simulink model "fskmodelo"  (R2015a)
settings: Solver=ode45  StartTime=0.0  StopTime=10.0  RelTol=1e-3
libraries: commdigbbndfm2 x2, commchan3 x1, commrandsrc2 x1, commsink2 x1
settings Model: Creator=francisco  LastModifiedBy=francisco

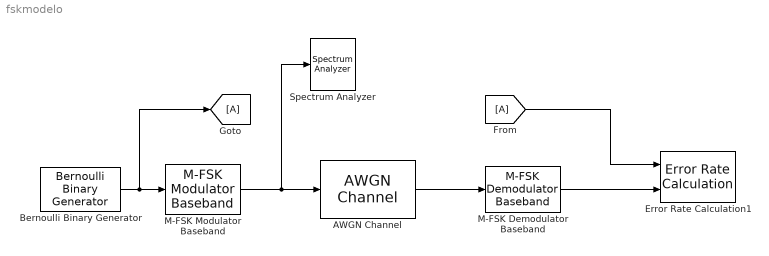
== system fskmodelo ==
  AWGN Channel : commchan3/AWGN Channel  InputProcessing=Columns as channels (frame based)  seed=67  noiseMode="Signal to noise ratio  (Eb/No)"  EbNodB=15  EsNodB=10  SNRdB=10  bitsPerSym=1  Ps=1  Tsym=1  variance=1
  Bernoulli Binary Generator : commrandsrc2/Bernoulli Binary Generator  P=0.5  seed=61  Ts=0.01  frameBased=off  sampPerFrame=1  orient=off  outDataType=double
  Error Rate Calculation1 : commsink2/Error Rate Calculation  N=0  st_delay=0  cp_mode=Entire frame  subframe=[]  PMode=Workspace  WsName=ErrorVec  RsMode2=off  stop=off  numErr=100  maxBits=1e6
  M-FSK Demodulator Baseband : commdigbbndfm2/M-FSK Demodulator Baseband  M=4  OutType=Integer  Dec=Gray  freqSep=100  numSamp=17  RateOptions=Enforce single-rate processing  outDataType=double
  M-FSK Modulator Baseband : commdigbbndfm2/M-FSK Modulator Baseband  M=4  InType=Integer  Enc=Gray  freqSep=100  phaseType=Continuous  numSamp=17  RateOptions=Enforce single-rate processing  outDataType=double
  Spectrum Analyzer : SpectrumAnalyzer
  wires:
  Bernoulli Binary Generator/1 -> [A], M-FSK Modulator Baseband/1
  M-FSK Demodulator Baseband/1 -> Error Rate Calculation1/2
  AWGN Channel/1 -> M-FSK Demodulator Baseband/1
  [A] -> Error Rate Calculation1/1
  M-FSK Modulator Baseband/1 -> Spectrum Analyzer/1, AWGN Channel/1
